simulink model "sl_R3GDL_RTB"  (Simulink 8.9)
settings: Solver=VariableStepAuto  StartTime=0.0  StopTime=tsim  MaxStep=1e-1  MinStep=1e-2  RelTol=1e-3  EnableMultiTasking=on
settings Model: Creator=Manuel G. Ortega  LastModifiedBy=Javi Gómez
settings OptimizationCC: ExpressionDepthLimit=2147483647
settings DebuggingCC: SolverPrmCheckMsg=warning
settings ConfigComp: CovSFcnEnable=off

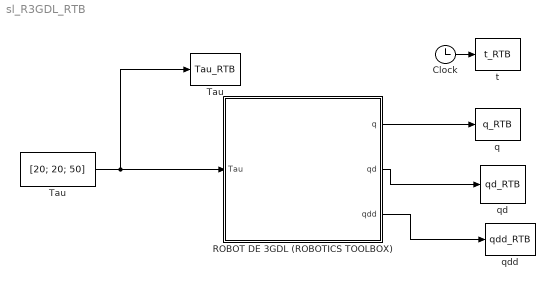
== system sl_R3GDL_RTB ==
  Clock : Clock
  ROBOT DE 3GDL (ROBOTICS TOOLBOX) : Subsystem
  Tau : Constant  Value=[20; 20; 50]  SampleTime=0
  "Tau " : ToWorkspace  VariableName=Tau_RTB  SampleTime=-1
  q : ToWorkspace  VariableName=q_RTB  SampleTime=-1
  qd : ToWorkspace  VariableName=qd_RTB  SampleTime=-1
  qdd : ToWorkspace  VariableName=qdd_RTB  SampleTime=-1
  t : ToWorkspace  VariableName=t_RTB  SampleTime=-1
  wires:
  Clock/1 -> t/1
  Tau/1 -> ROBOT DE 3GDL (ROBOTICS TOOLBOX)/1(Tau), "Tau "/1
  ROBOT DE 3GDL (ROBOTICS TOOLBOX)/1(q) -> q/1
  ROBOT DE 3GDL (ROBOTICS TOOLBOX)/2(qd) -> qd/1
  ROBOT DE 3GDL (ROBOTICS TOOLBOX)/3(qdd) -> qdd/1

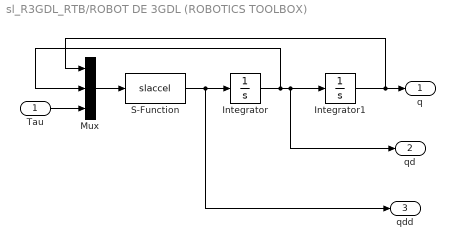
== system sl_R3GDL_RTB/ROBOT DE 3GDL (ROBOTICS TOOLBOX) ==
  Tau : Inport
  Integrator : Integrator  InitialCondition=[0; 0; 0]
  Integrator1 : Integrator  InitialCondition=[0; 0; 0]
  Mux : Mux  Inputs=3
  S-Function : S-Function  FunctionName=slaccel  Parameters=R3GDL  SFunctionDeploymentMode=off  EnableBusSupport=off
  q : Outport
  qd : Outport  Port=2
  qdd : Outport  Port=3
  wires:
  S-Function/1 -> Integrator/1, qdd/1
  Integrator/1 -> Integrator1/1, qd/1, Mux/2
  Integrator1/1 -> Mux/1, q/1
  Mux/1 -> S-Function/1
  Tau/1 -> Mux/3
